simulink model "am_sys2"  (Simulink 3.00)
settings: Solver=ode45  StartTime=0.0  StopTime=999999  MaxStep=0.001  RelTol=1e-3  AbsTol=1e-3
undefined symbols (not defined in the file): at, bt, ct, dt, offset
settings Model: SaveTime=off  SaveOutput=off

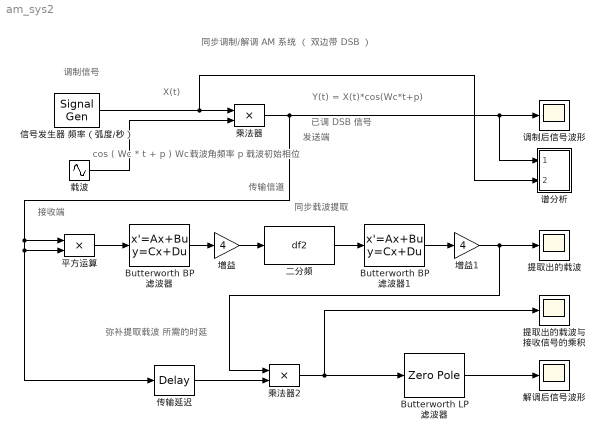
== system am_sys2 ==
  note: 同步调制/解调 AM 系统 （ 双边带 DSB ）
  note: 同步载波提取
  note: 接收端
  note: 已调 DSB 信号
  note: 发送端
  note: Y(t) = X(t)*cos(Wc*t+p)
  note: X(t)
  note: 调制信号
  note: 弥补提取载波
      | 所需的时延
  note: cos ( Wc * t + p )
      | Wc 载波角频率
      | p 载波初始相位
  note: 传输信道
  Butterworth BP 滤波器 : StateSpace  A=at  B=bt  C=ct  D=dt  X0=0  mask(buttap,lp2bp){@1=200, @2=10, @3=4}
      mask prompts: @1 "Center frequency (rad/sec)"; @2 "Bandwidth (rad/sec):"; @3 "Order"
      mask help:
      | Analog Butterworth band pass filter.
      |
      | (Requires Signal Processing Toolbox)
      mask init:
      | [at,bt,ct,dt,w,mag]=filtm('buttap','lp2bp',@1,@2,50,@3);
      mask Help: Butterworth band pass filter using MATLAB's butter and lp2bp command.
      mask Display: plot(w,mag)
  Butterworth BP 滤波器1 : StateSpace  A=at  B=bt  C=ct  D=dt  X0=0  mask(buttap,lp2bp){@1=100, @2=10, @3=4}
      mask prompts: @1 "Center frequency (rad/sec)"; @2 "Bandwidth (rad/sec):"; @3 "Order"
      mask help:
      | Analog Butterworth band pass filter.
      |
      | (Requires Signal Processing Toolbox)
      mask init:
      | [at,bt,ct,dt,w,mag]=filtm('buttap','lp2bp',@1,@2,50,@3);
      mask Help: Butterworth band pass filter using MATLAB's butter and lp2bp command.
      mask Display: plot(w,mag)
  Butterworth LP 滤波器 : ZeroPole  Zeros=z  Poles=p  Gain=k  mask(buttap){@1=10, @2=4}
      mask prompts: @1 "Cutoff frequency (rad/sec)"; @2 "Order"
      mask help:
      | Analog Butterworth low pass filter.
      |
      | (Requires Signal Processing Toolbox)
      mask init:
      | [z,p,k]=buttap(@2); z=@1*z; p=@1*p; k=real(prod(-p)); [num,den]=zp2tf(z,p,k); w=logspace(log10(@1/10),log10(10*@1),20); h=freqs(num,den,w);
      mask Help: Butterworth low pass filter using MATLAB's butter command.
      mask Display: plot(20*log10(w),20*log10(abs(h)))
  乘法器 : Product  Inputs=2  SaturateOnIntegerOverflow=on
      mask Type: 乘法器
      mask Description: 乘法器
      mask Display: plot([0 1],[1 0],[0 1],[0 1]);
  乘法器2 : Product  Inputs=2  SaturateOnIntegerOverflow=on
      mask Type: 乘法器
      mask Description: 乘法器
      mask Display: plot([0 1],[1 0],[0 1],[0 1]);
  传输延迟 : TransportDelay  DelayTime=0.09  InitialInput=0  BufferSize=1024
  调制后信号波形 : Scope
      settings: TimeRange=1.000000  YMin=-2  YMax=2  SaveToWorkspace=off  SaveName=ScopeData  DataFormat=Matrix
  二分频 : MATLABFcn  MATLABFcn=df2  OutputWidth=-1  OutputSignalType=auto
      mask Type: 分频器
      mask Description: 二分频器
      mask Display: disp('Frequency\n—————\n2')
  解调后信号波形 : Scope
      settings: TimeRange=1.000000  YMin=-3  YMax=3  SaveToWorkspace=off  SaveName=ScopeData  DataFormat=Matrix
  平方运算 : Product  Inputs=2  SaturateOnIntegerOverflow=on
      mask Type: 乘法器
      mask Description: 乘法器
      mask Display: plot([0 1],[1 0],[0 1],[0 1]);
  谱分析 : Subsystem  mask(Spectrum analyzer.){@1=512, @2=512, @3=64, @4=0.001}
      mask prompts: @1 "Length of buffer:"; @2 "Number of points for fft:"; @3 "Plot after how many points:"; @4 "Sample time:"
      mask help:
      | Spectrum analyser using graph window.
      | Hook input 1 to system input.
      | Hook input 2 to system output.
      mask init:
      | npts=@1; fftpts=@2; HowOften=@3; ts=@4(1); if length(@4) > 1, offset = @4(2), else, offset = 0; end
      mask Help: Hook the system's input to the first port of this block and the system's output to second port. Results are displayed as the frequency response of this system. Use signals with high harmonic content for best results.
      mask Display: plot(0,0,100,100,[11,93,93,11,11],[90,90,40,40,90],[90,80,72,64,55,45,41,36,20],[50,50,52,59,67,75,78,80,80])
  提取出的载波 : Scope
      settings: TimeRange=1.000000  YMin=-4  YMax=4  SaveToWorkspace=off  SaveName=ScopeData  DataFormat=Matrix
  提取出的载波与 接收信号的乘积 : Scope
      settings: TimeRange=1.000000  YMin=-4  YMax=4  SaveToWorkspace=off  SaveName=ScopeData  DataFormat=Matrix
  信号发生器 频率（弧度/秒） : SignalGenerator  WaveForm=sine  Amplitude=1.000000  Frequency=10.000000  Units=rad/sec
  载波 : Sin  Amplitude=1  Frequency=100  Phase=0  SampleTime=0.001
  增益 : Gain  Gain=4  SaturateOnIntegerOverflow=on
  增益1 : Gain  Gain=4  SaturateOnIntegerOverflow=on
  wires:
  载波/1 -> 乘法器/2
  平方运算/1 -> Butterworth BP 滤波器/1
  Butterworth BP 滤波器/1 -> 增益/1
  增益/1 -> 二分频/1
  二分频/1 -> Butterworth BP 滤波器1/1
  Butterworth BP 滤波器1/1 -> 增益1/1
  传输延迟/1 -> 乘法器2/2
  增益1/1 -> 提取出的载波/1, 乘法器2/1
  Butterworth LP 滤波器/1 -> 解调后信号波形/1
  乘法器2/1 -> Butterworth LP 滤波器/1, 提取出的载波与 接收信号的乘积/1
  乘法器/1 -> 传输延迟/1, 平方运算/2, 平方运算/1, 调制后信号波形/1, 谱分析/1(system input)
  信号发生器 频率（弧度/秒）/1 -> 乘法器/1, 谱分析/2(system output)

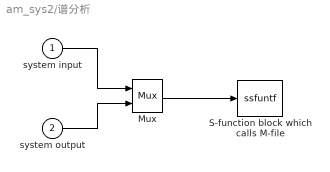
== system am_sys2/谱分析 ==
  system input : Inport  Port=1  PortWidth=-1  SampleTime=-1  DataType=auto
      settings: SignalType=auto
  system output : Inport  Port=2  PortWidth=-1  SampleTime=-1  DataType=auto
      settings: SignalType=auto
  Mux : Mux  Inputs=2
      settings: DisplayOption=none
  S-function block which calls M-file : S-Function  FunctionName=ssfuntf  Parameters=fftpts,npts,HowOften,offset,ts,0  PortCounts=[]  SFunctionModules=''
  wires:
  system output/1 -> Mux/2
  system input/1 -> Mux/1
  Mux/1 -> S-function block which calls M-file/1
